simulink model "SchlossBox"  (R2017b)
settings: Solver=FixedStepAuto  StartTime=0.0  StopTime=10.0  RelTol=1e-3
PreLoadFcn:
  | waijung.modelPreload; % Required for working with Waijung Blockset. Do not remove.
undefined symbols (not defined in the file): Blocking, HSEOSC, Link, LQFP100, Non, ST, STM32F407VG
libraries: stm32f4_canbus_lib x8, simulink x6, stm32f4_io_lib x4, stm32f4_device_config_lib x1
CloseFcn:
  | waijung.modelClose; % Required for working with Waijung Blockset. Do not remove.
settings Model: Creator=labuser  LastModifiedBy=labuser
settings OptimizationCC: DefaultParameterBehavior=Inlined  PassReuseOutputArgsAs=Individual arguments
settings DebuggingCC: ParameterTunabilityLossMsg=error
settings HardwareCC: ProdBitPerPointer=32  ProdBitPerSizeT=32  ProdBitPerPtrDiffT=32  ProdLargestAtomicFloat=None  ProdIntDivRoundTo=Undefined  ProdWordSize=32  ProdHWDeviceType=ARM Compatible->Cortex - M4  TargetEndianess=LittleEndian  TargetHWDeviceType=ARM Compatible->Cortex - M4
settings SFSimCC: MATLABDynamicMemAlloc=off
settings RTWCC: SystemTargetFile=stm32f4.tlc  GenerateMakefile=off  TemplateMakefile=ert_default_tmf  Description=STM32F4 Target  GenerateReport=on  IncludeHyperlinkInReport=on  LaunchReport=on  GenerateTraceInfo=on  GenerateTraceReport=on  GenerateTraceReportSl=on  GenerateTraceReportSf=on  GenerateTraceReportEml=on
settings CodeAppCC: ForceParamTrailComments=on  IgnoreCustomStorageClasses=off  OperatorAnnotations=on  SimulinkDataObjDesc=on  SFDataObjDesc=on  InsertBlockDesc=on
settings STFCustomTargetCC: TargetLangStandard=C99 (ISO)  MultiwordLength=256  ModelReferenceCompliant=off  CombineOutputUpdateFcns=on  ERTCustomFileBanners=on  SupportContinuousTime=off  SupportNonInlinedSFcns=off  RemoveResetFunc=on  MATLABClassNameForMDSCustomization=Simulink.SoftwareTarget.ERTCustomization  GRTInterface=off  SystemTargetFile=stm32f4.tlc
settings ERTTargetCC: TargetLangStandard=C99 (ISO)  ModelReferenceCompliant=off  ParMdlRefBuildCompliant=off  CompOptLevelCompliant=off  ConcurrentExecutionCompliant=off  ModelStepFunctionPrototypeControlCompliant=off  CPPClassGenCompliant=off  UseToolchainInfoCompliant=off  InlinedParameterPlacement=NonHierarchical  ERTSrcFileBannerTemplate=stm32f4_code_template.cgt  ERTHdrFileBannerTemplate=stm32f4_code_template.cgt  ERTDataSrcFileTemplate=stm32f4_code_template.cgt  ERTDataHdrFileTemplate=stm32f4_code_template.cgt  ERTCustomFileTemplate=stm32f4_file_process.tlc

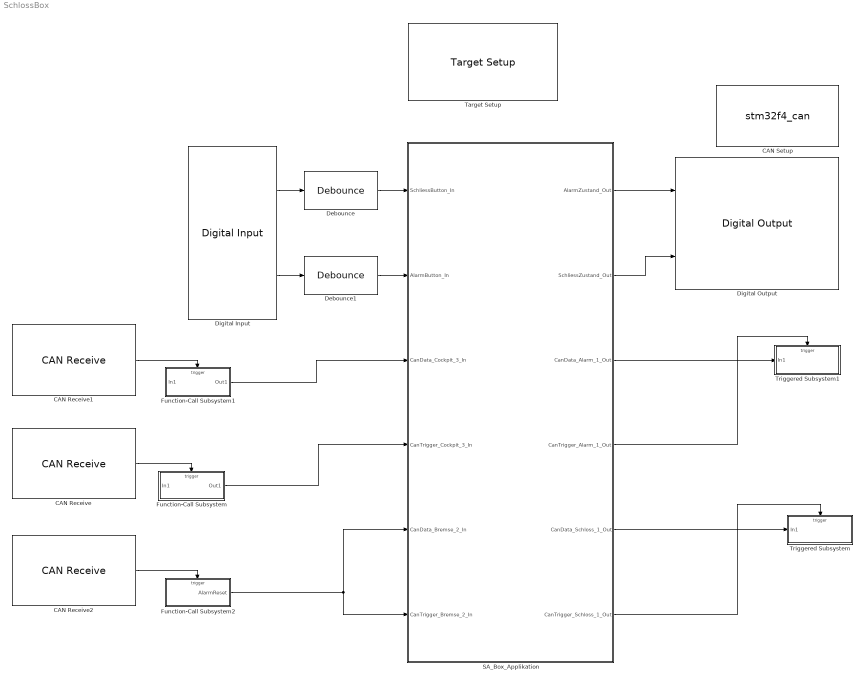
== system SchlossBox ==
  CAN Receive : stm32f4_canbus_lib/CAN Receive  conf=Rx  canmodule=1  idtype=Standard  filtertype=Specific  id=18  idmask=0  enableisr=on  usedlc=off  datatype=single  data0type=uint32  data1type=uint32  data2type=Not used  data3type=Not used  data4type=Not used  data5type=Not used  data6type=Not used  data7type=Not used  buffersize=8  sampletime=-1  sampletimestr=-1  blockid=CANReceive  inputarray=[]  inputlabelarray={}  outputarray=[7]  outputlabelarray={'Call ISR' }  compat=0  confstr="[\"Standard\",\"Specific\",\"18\",\"0\",\"off\",\"uint32\",\"uint32\",\"Not used\",\"Not used\",\"Not used\",\"Not used\",\"Not used\",\"Not used\",\"8\",\"240\",\"0\",\"FFE0\",\"4\"]"
      settings: SourceProductName=Waijung Blockset
  CAN Receive1 : stm32f4_canbus_lib/CAN Receive  conf=Rx  canmodule=1  idtype=Standard  filtertype=Specific  id=18  idmask=0  enableisr=on  usedlc=off  datatype=single  data0type=uint32  data1type=uint32  data2type=Not used  data3type=Not used  data4type=Not used  data5type=Not used  data6type=Not used  data7type=Not used  buffersize=8  sampletime=-1  sampletimestr=-1  blockid=CANReceive1  inputarray=[]  inputlabelarray={}  outputarray=[7]  outputlabelarray={'Call ISR' }  compat=0  confstr="[\"Standard\",\"Specific\",\"18\",\"0\",\"off\",\"uint32\",\"uint32\",\"Not used\",\"Not used\",\"Not used\",\"Not used\",\"Not used\",\"Not used\",\"8\",\"240\",\"0\",\"FFE0\",\"4\"]"
      settings: SourceProductName=Waijung Blockset
  CAN Receive2 : stm32f4_canbus_lib/CAN Receive  conf=Rx  canmodule=1  idtype=Standard  filtertype=Specific  id=12  idmask=0  enableisr=on  usedlc=off  datatype=single  data0type=uint32  data1type=uint32  data2type=Not used  data3type=Not used  data4type=Not used  data5type=Not used  data6type=Not used  data7type=Not used  buffersize=8  sampletime=-1  sampletimestr=-1  blockid=CANReceive1  inputarray=[]  inputlabelarray={}  outputarray=[7]  outputlabelarray={'Call ISR' }  compat=0  confstr="[\"Standard\",\"Specific\",\"12\",\"0\",\"off\",\"uint32\",\"uint32\",\"Not used\",\"Not used\",\"Not used\",\"Not used\",\"Not used\",\"Not used\",\"8\",\"180\",\"0\",\"FFE0\",\"4\"]"
      settings: SourceProductName=Waijung Blockset
  CAN Setup : S-Function  FunctionName=stm32f4_can  Parameters=conf,canmodule,0,inputarray,outputarray,'','',confstr,sampletime,sampletimestr,blockid  SFunctionDeploymentMode=off  EnableBusSupport=off  mask(stm32f4_can){conf=Setup, canmodule=1, advance=off, bitrate_select=125000, sjw=1tq, bs1=14tq, bs2=6tq, timingconf=Prescaler, brp=16, bitrate=125000, tq=3.8095e-07, autoretransmission=Disable, remaptxpin=D1, remaprxpin=D0, sampletime=0.01, sampletimestr=-1, blockid=CANSetup, inputarray=[], inputlabelarray={}, outputarray=[], outputlabelarray={}, compat=0, confstr=["125000","16","D","1","D","0","1tq","14tq","6tq","ENABLE"], presc=16, txportstr=D, txpinstr=1, rxportstr=D, rxpinstr=0, lastmodule=1}
      mask prompts: conf "Configuration"; canmodule "CAN Module"; advance "Advance configuration"; bitrate_select "Baud rate (bps)"; sjw "Resync Jump Width (SJW)"; bs1 "Bit segment 1 (BS1) + PROP_SEG"; bs2 "Bit segment 2 (BS2)"; timingconf "Adjust"; brp "Baud rate prescaler (BRP)"; bitrate "Baud rate (bps)"; tq "Time Quantum (Second), tq"; autoretransmission "Auto Re-transmission"; remaptxpin "CAN Tx pin"; remaprxpin "CAN Rx pin"; sampletime "Sample time (sec)"; sampletimestr "Compiled sample time (sec) in string"; inputarray "Input port"; inputlabelarray "Input port label"; outputarray "Output port"; outputlabelarray "Output port label"; compat "Compatibility (Reserved for future use)"; confstr "Configuration String"; presc "Prescale"; txportstr "Tx port string"; txpinstr "Tx pin string"; rxportstr "Rx port string"; rxpinstr "Rx pin string"; lastmodule "Last module selected"
      mask help:
      | This block setups CAN Module.
      |
      | Auto Re-transmission,
      |  - Enable: The CAN hardware will automatically retransmit the message until it has been
      | successfully transmitted according to the CAN standard.
      |  - Disable: A message will be transmitted only once, independently of the transmission result
      | (successful, error or arbitration lost).
      mask init:
      | stm32f4_can_callback('init');
      mask Help: web(fullfile(waijungdocroot,'stm32f4_can_setup.htm'), '-browser')
      mask TypeOptions conf: Setup
      mask TypeOptions canmodule: 1 | 2
      mask Callback canmodule: stm32f4_can_callback('canmodule');
      mask Callback advance: stm32f4_can_callback('advance');
      mask TypeOptions bitrate_select: 125000 | 250000 | 500000 | 1000000
      mask Callback bitrate_select: stm32f4_can_callback('bitrate_select');
      mask TypeOptions sjw: 1tq | 2tq | 3tq | 4tq
      mask TypeOptions bs1: 1tq | 2tq | 3tq | 4tq | 5tq | 6tq | 7tq | 8tq | 9tq | 10tq | 11tq | 12tq | 13tq | 14tq | 15tq | 16tq
      mask Callback bs1: stm32f4_can_callback('timingconf');
      mask TypeOptions bs2: 1tq | 2tq | 3tq | 4tq | 5tq | 6tq | 7tq | 8tq
      mask Callback bs2: stm32f4_can_callback('timingconf');
      mask TypeOptions timingconf: Prescaler | Baudrate
      mask Callback timingconf: stm32f4_can_callback('timingconf');
      mask Callback brp: stm32f4_can_callback('timingconf');
      mask Callback bitrate: stm32f4_can_callback('timingconf');
      mask TypeOptions autoretransmission: Enable | Disable
      mask TypeOptions remaptxpin: Not used | A12 | B9 | D1
      mask Callback remaptxpin: stm32f4_can_callback('remaptxpin');
      mask TypeOptions remaprxpin: Not used | A11 | B8 | D0
      mask Callback remaprxpin: stm32f4_can_callback('remaprxpin');
      mask Callback sampletime: stm32f4_can_callback('sampletime');
      mask Callback sampletimestr: stm32f4_can_callback('sampletimestr');
      mask Callback blockid: stm32f4_can_callback('blockid');
      mask Display: text(0.5, 0.5, 'CAN1_Setup\nSpeed (bps): 125000\nTx/Rx pin: D1/D0','ver','middle','hor','center');
  Debounce : stm32f4_io_lib/Debounce  mode=Normal  prescale=4  debounce=4
      settings: SourceProductName=Waijung Blockset
  Debounce1 : stm32f4_io_lib/Debounce  mode=Normal  prescale=4  debounce=4
      settings: SourceProductName=Waijung Blockset
  Digital Input : stm32f4_io_lib/Digital Input  port=C  speed=100  porttype=None  porttypestr=NOPULL  use_pin0=on  use_pin1=on  use_pin2=off  use_pin3=off  use_pin4=off  use_pin5=off  use_pin6=off  use_pin7=off  use_pin8=off  use_pin9=off  use_pin10=off  use_pin11=off  use_pin12=off  use_pin13=off  use_pin14=off  use_pin15=off  pinstr=GPIO_Pin_0 | GPIO_Pin_1  usedpinarray="[1  1  0  0  0  0  0  0  0  0  0  0  0  0  0  0]"  bitbandingstr=|  sampletime=-1  sampletimestr=-1  blockid=DigitalInput  enablecustomportlabel=off  glabalinit=off  cinputportlabel=In1, In2  coutputportlabel=Out1, Out2
      | #define DigitalInput_C0 Peripheral_BB(GPIOC->IDR, 0)  /* Output pin */
      | #define DigitalInput_C1 Peripheral_BB(GPIOC->IDR, 1)  /* Output pin */
      settings: SourceProductName=Waijung Blockset
  Digital Output : stm32f4_io_lib/Digital Output  use_bitband=on  port=C  speed=100  porttype=Push Pull  porttypestr=PP  use_pin0=off  use_pin1=off  use_pin2=on  use_pin3=on  use_pin4=off  use_pin5=off  use_pin6=off  use_pin7=off  use_pin8=off  use_pin9=off  use_pin10=off  use_pin11=off  use_pin12=off  use_pin13=off  use_pin14=off  use_pin15=off  pinstr=GPIO_Pin_2 | GPIO_Pin_3  usedpinarray="[0  0  1  1  0  0  0  0  0  0  0  0  0  0  0  0]"  bitbandingstr=|  sampletime=-1  sampletimestr=-1  blockid=DigitalOutput  enablecustomportlabel=off  globalinit=off  cinputportlabel=In1, In2  coutputportlabel=0
      | #define DigitalOutput_C2 Peripheral_BB(GPIOC->ODR, 2)  /* Output pin */
      | #define DigitalOutput_C3 Peripheral_BB(GPIOC->ODR, 3)  /* Output pin */
      settings: SourceProductName=Waijung Blockset
  Function-Call Subsystem : Subsystem  TreatAsAtomicUnit=on
  Function-Call Subsystem1 : Subsystem  TreatAsAtomicUnit=on
  Function-Call Subsystem2 : Subsystem  TreatAsAtomicUnit=on
  SA_Box_Applikation : Subsystem
  Target Setup : stm32f4_device_config_lib/Target Setup  Priority=100  compiler=GNU ARM  previous_compiler=GNU ARM  mcu=STM32F407VG (LQFP100)  mcustr=STM32F407VG  clockconfig=HSEOSC-8MHz  system_stm32f4xx_c_path=C:\waijung17_03a\targets\stm32f4_target\stm32f4\utils\system_stm32f4xx_default\STM32F40_41xxx\hseosc8mhz  showmemoryconfiguration=off  stacksize=0x2000  heapsize=0x2000  enableautocompiledownload=on  fullchiperase=off  programmerinterface=ST-Link  editctrlstr=on  compilercontrolstr=$(patsubst %, -I%, .) -mcpu=cortex-m4 -mthumb -mthumb-interwork -mfloat-abi=hard -mfpu=fpv4-sp-d16 -ffast-math -Wall -Wextra -Ofast  assemblercontrolstr=$(patsubst %, -I%, .) -mcpu=cortex-m4 -mthumb -mthumb-interwork -mfloat-abi=hard -mfpu=fpv4-sp-d16 -ffast-math -Wall -Wextra -Ofast -Wa,-amhls=$(<:.s=.lst) -D__STACK_SIZE=$(STACK_SIZE) -D__HEAP_SIZE=$(HEAP_SIZE)  linkercontrolstr=-T$(LD_SCRIPT) -g -Wl,-Map=$(MAP),--cref,--no-warn-mismatch -mcpu=cortex-m4 -mthumb -mthumb-interwork -mfloat-abi=hard -mfpu=fpv4-sp-d16 -specs=nosys.specs  runafterdownload=on  execprofile=None  profileruart=3  profilerbaud=500000  profilertxpin=D8  profilerinitstr=0.01,168000000,1680000,500000,0  manualsetsampletime=off  sampletime=0.01  blockid=TargetSetup  systickreloadvalue=1680000  hseval=8000000  lastprofileruart=3  hclk=168000000  flashorigin=0x8000000  flashlength=1024k  ramorigin=0x20000000  ramlength=128k  useextram=off
      settings: SourceProductName=Waijung Blockset
  Triggered Subsystem : Subsystem  TreatAsAtomicUnit=on
  Triggered Subsystem1 : Subsystem  TreatAsAtomicUnit=on
  wires:
  Function-Call Subsystem2/1(AlarmReset) -> SA_Box_Applikation/5(CanData_Bremse_2_In), SA_Box_Applikation/6(CanTrigger_Bremse_2_In)
  SA_Box_Applikation/5(CanData_Schloss_1_Out) -> Triggered Subsystem/1(In1)
  CAN Receive/1 -> Function-Call Subsystem/Trigger
  Function-Call Subsystem/1(Out1) -> SA_Box_Applikation/4(CanTrigger_Cockpit_3_In)
  CAN Receive1/1 -> Function-Call Subsystem1/Trigger
  Function-Call Subsystem1/1(Out1) -> SA_Box_Applikation/3(CanData_Cockpit_3_In)
  Digital Input/2 -> Debounce1/1
  SA_Box_Applikation/3(CanData_Alarm_1_Out) -> Triggered Subsystem1/1(In1)
  SA_Box_Applikation/2(SchliessZustand_Out) -> Digital Output/2
  SA_Box_Applikation/1(AlarmZustand_Out) -> Digital Output/1
  Digital Input/1 -> Debounce/1
  Debounce/1 -> SA_Box_Applikation/1(SchliessButton_In)
  Debounce1/1 -> SA_Box_Applikation/2(AlarmButton_In)
  SA_Box_Applikation/4(CanTrigger_Alarm_1_Out) -> Triggered Subsystem1/Trigger
  SA_Box_Applikation/6(CanTrigger_Schloss_1_Out) -> Triggered Subsystem/Trigger
  CAN Receive2/1 -> Function-Call Subsystem2/Trigger

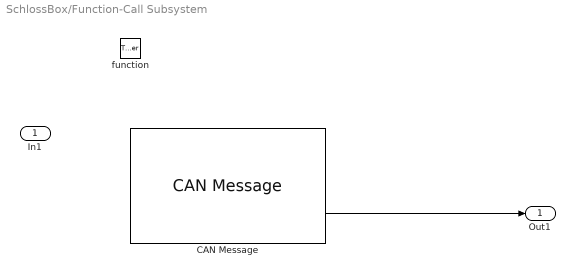
== system SchlossBox/Function-Call Subsystem ==
  In1 : Inport
  function : TriggerPort  TriggerType=function-call  VariantControl=Variant
  CAN Message : stm32f4_canbus_lib/CAN Message  conf=Msg  canmodule=1  usedlc=off  datatype=double  data0type=uint8  data1type=Not used  data2type=Not used  data3type=Not used  data4type=Not used  data5type=Not used  data6type=Not used  data7type=Not used  sampletime=-1  sampletimestr=-1  blockid=FunctionCallSubsystemCANMessage  inputarray=[]  inputlabelarray={}  outputarray=[ 7, 3]  outputlabelarray={'ID', 'D0 (uint8)' }  compat=0  confstr="[\"off\",\"uint8\",\"Not used\",\"Not used\",\"Not used\",\"Not used\",\"Not used\",\"Not used\",\"Not used\"]"
      settings: SourceProductName=Waijung Blockset
  Out1 : Outport
  wires:
  CAN Message/2 -> Out1/1

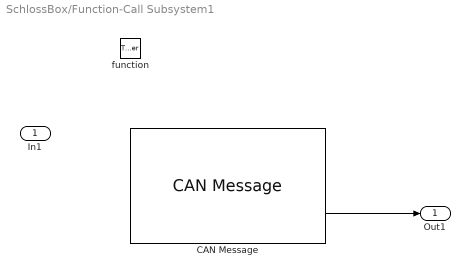
== system SchlossBox/Function-Call Subsystem1 ==
  In1 : Inport
  function : TriggerPort  TriggerType=function-call  VariantControl=Variant
  CAN Message : stm32f4_canbus_lib/CAN Message  conf=Msg  canmodule=1  usedlc=off  datatype=double  data0type=uint8  data1type=Not used  data2type=Not used  data3type=Not used  data4type=Not used  data5type=Not used  data6type=Not used  data7type=Not used  sampletime=-1  sampletimestr=-1  blockid=FunctionCallSubsystem1CANMessage  inputarray=[]  inputlabelarray={}  outputarray=[ 7, 3]  outputlabelarray={'ID', 'D0 (uint8)' }  compat=0  confstr="[\"off\",\"uint8\",\"Not used\",\"Not used\",\"Not used\",\"Not used\",\"Not used\",\"Not used\",\"Not used\"]"
      settings: SourceProductName=Waijung Blockset
  Out1 : Outport
  wires:
  CAN Message/2 -> Out1/1

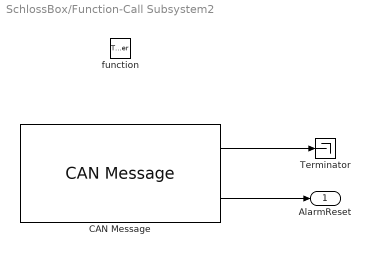
== system SchlossBox/Function-Call Subsystem2 ==
  function : TriggerPort  TriggerType=function-call  VariantControl=Variant
  CAN Message : stm32f4_canbus_lib/CAN Message  conf=Msg  canmodule=1  usedlc=off  datatype=double  data0type=uint8  data1type=Not used  data2type=Not used  data3type=Not used  data4type=Not used  data5type=Not used  data6type=Not used  data7type=Not used  sampletime=-1  sampletimestr=-1  blockid=FunctionCallSubsystem1CANMessage  inputarray=[]  inputlabelarray={}  outputarray=[ 7, 3]  outputlabelarray={'ID', 'D0 (uint8)' }  compat=0  confstr="[\"off\",\"uint8\",\"Not used\",\"Not used\",\"Not used\",\"Not used\",\"Not used\",\"Not used\",\"Not used\"]"
      settings: SourceProductName=Waijung Blockset
  Terminator : Terminator
  AlarmReset : Outport
  wires:
  CAN Message/1 -> Terminator/1
  CAN Message/2 -> AlarmReset/1

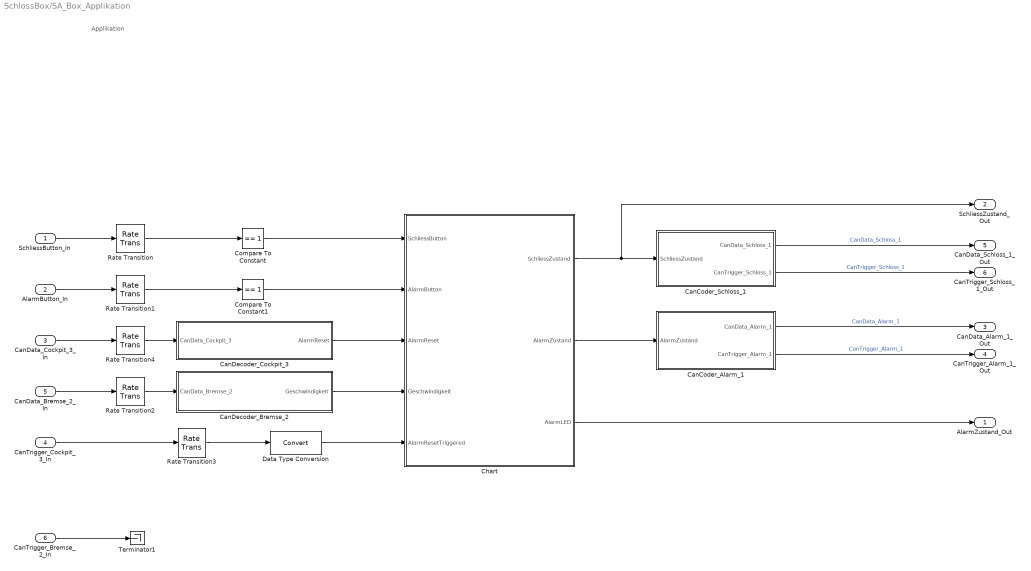
== system SchlossBox/SA_Box_Applikation ==
  note: Applikation
  SchliessButton_In : Inport
  AlarmButton_In : Inport  Port=2
  CanData_Cockpit_3_In : Inport  Port=3
  CanTrigger_Cockpit_3_In : Inport  Port=4
  CanData_Bremse_2_In : Inport  Port=5
  CanTrigger_Bremse_2_In : Inport  Port=6
  CanCoder_Alarm_1 : Subsystem
  CanCoder_Schloss_1 : Subsystem
  CanDecoder_Bremse_2 : Subsystem
  CanDecoder_Cockpit_3 : Subsystem
  Chart : Stateflow chart  TreatAsAtomicUnit=on
  Compare To Constant : simulink/Logic and Bit Operations/Compare To Constant  relop===  const=1  OutDataTypeStr=uint8
  Compare To Constant1 : simulink/Logic and Bit Operations/Compare To Constant  relop===  const=1  OutDataTypeStr=uint8
  Data Type Conversion : DataTypeConversion
  Rate Transition{,1..4} (5 alike) : RateTransition  Deterministic=off  OutPortSampleTimeOpt=Inherit
  Terminator1 : Terminator
  AlarmZustand_Out : Outport
  SchliessZustand_Out : Outport  Port=2
  CanData_Alarm_1_Out : Outport  Port=3
  CanTrigger_Alarm_1_Out : Outport  Port=4
  CanData_Schloss_1_Out : Outport  Port=5
  CanTrigger_Schloss_1_Out : Outport  Port=6
  wires:
  CanCoder_Schloss_1/1(CanData_Schloss_1) -> CanData_Schloss_1_Out/1  "CanData_Schloss_1"
  CanCoder_Alarm_1/1(CanData_Alarm_1) -> CanData_Alarm_1_Out/1  "CanData_Alarm_1"
  CanCoder_Alarm_1/2(CanTrigger_Alarm_1) -> CanTrigger_Alarm_1_Out/1  "CanTrigger_Alarm_1"
  CanCoder_Schloss_1/2(CanTrigger_Schloss_1) -> CanTrigger_Schloss_1_Out/1  "CanTrigger_Schloss_1"
  CanDecoder_Cockpit_3/1(AlarmReset) -> Chart/3(AlarmReset)
  CanDecoder_Bremse_2/1(Geschwindigkeit) -> Chart/4(Geschwindigkeit)
  Chart/2(AlarmZustand) -> CanCoder_Alarm_1/1(AlarmZustand)
  CanData_Cockpit_3_In/1 -> Rate Transition4/1
  SchliessButton_In/1 -> Rate Transition/1
  CanData_Bremse_2_In/1 -> Rate Transition2/1
  AlarmButton_In/1 -> Rate Transition1/1
  CanTrigger_Bremse_2_In/1 -> Terminator1/1
  Chart/3(AlarmLED) -> AlarmZustand_Out/1
  Chart/1(SchliessZustand) -> SchliessZustand_Out/1, CanCoder_Schloss_1/1(SchliessZustand)
  Rate Transition4/1 -> CanDecoder_Cockpit_3/1(CanData_Cockpit_3)
  Rate Transition2/1 -> CanDecoder_Bremse_2/1(CanData_Bremse_2)
  Rate Transition3/1 -> Data Type Conversion/1
  CanTrigger_Cockpit_3_In/1 -> Rate Transition3/1
  Data Type Conversion/1 -> Chart/5(AlarmResetTriggered)
  Rate Transition/1 -> Compare To Constant/1
  Rate Transition1/1 -> Compare To Constant1/1
  Compare To Constant/1 -> Chart/1(SchliessButton)
  Compare To Constant1/1 -> Chart/2(AlarmButton)

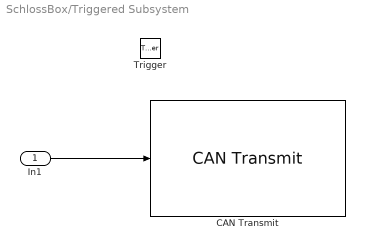
== system SchlossBox/Triggered Subsystem ==
  In1 : Inport
  Trigger : TriggerPort  VariantControl=Variant
  CAN Transmit : stm32f4_canbus_lib/CAN Transmit  conf=Tx  canmodule=1  transfer=Non-Blocking  timeout=0.005  idtype=Standard  specificid=on  id=25  specificdlc=on  dlc=2  enablestatus=off  datatype=single  data0type=int16  data1type=Not used  data2type=Not used  data3type=Not used  data4type=Not used  data5type=Not used  data6type=Not used  data7type=Not used  inputarray=[ 4]  inputlabelarray={ 'D0 (int16)' }  outputarray=[]  outputlabelarray={}  sampletime=-1  sampletimestr=-1  blockid=TriggeredSubsystemCANTransmit  compat=0  confstr="[\"Non-Blocking\",\"0.005\",\"Standard\",\"on\",\"25\",\"on\",\"2\",\"off\",\"int16\",\"Not used\",\"Not used\",\"Not used\",\"Not used\",\"Not used\",\"Not used\",\"Not used\"]"
      settings: SourceProductName=Waijung Blockset
  wires:
  In1/1 -> CAN Transmit/1

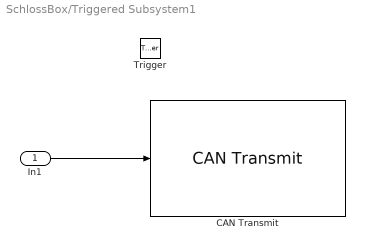
== system SchlossBox/Triggered Subsystem1 ==
  In1 : Inport
  Trigger : TriggerPort  VariantControl=Variant
  CAN Transmit : stm32f4_canbus_lib/CAN Transmit  conf=Tx  canmodule=1  transfer=Non-Blocking  timeout=0.005  idtype=Standard  specificid=on  id=20  specificdlc=on  dlc=2  enablestatus=off  datatype=single  data0type=int16  data1type=Not used  data2type=Not used  data3type=Not used  data4type=Not used  data5type=Not used  data6type=Not used  data7type=Not used  inputarray=[ 4]  inputlabelarray={ 'D0 (int16)' }  outputarray=[]  outputlabelarray={}  sampletime=-1  sampletimestr=-1  blockid=TriggeredSubsystem1CANTransmit  compat=0  confstr="[\"Non-Blocking\",\"0.005\",\"Standard\",\"on\",\"20\",\"on\",\"2\",\"off\",\"int16\",\"Not used\",\"Not used\",\"Not used\",\"Not used\",\"Not used\",\"Not used\",\"Not used\"]"
      settings: SourceProductName=Waijung Blockset
  wires:
  In1/1 -> CAN Transmit/1

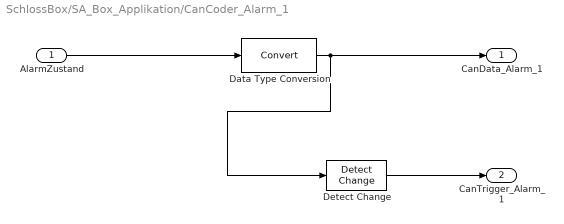
== system SchlossBox/SA_Box_Applikation/CanCoder_Alarm_1 ==
  AlarmZustand : Inport
  Data Type Conversion : DataTypeConversion
  Detect Change : simulink/Logic and Bit Operations/Detect Change  vinit=0  OutDataTypeStr=uint8
  CanData_Alarm_1 : Outport
  CanTrigger_Alarm_1 : Outport  Port=2
  wires:
  Detect Change/1 -> CanTrigger_Alarm_1/1
  AlarmZustand/1 -> Data Type Conversion/1
  Data Type Conversion/1 -> Detect Change/1, CanData_Alarm_1/1

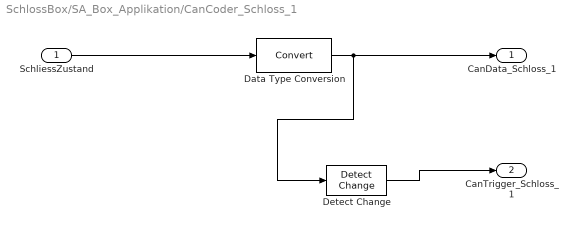
== system SchlossBox/SA_Box_Applikation/CanCoder_Schloss_1 ==
  SchliessZustand : Inport
  Data Type Conversion : DataTypeConversion
  Detect Change : simulink/Logic and Bit Operations/Detect Change  vinit=0  OutDataTypeStr=uint8
  CanData_Schloss_1 : Outport
  CanTrigger_Schloss_1 : Outport  Port=2
  wires:
  SchliessZustand/1 -> Data Type Conversion/1
  Data Type Conversion/1 -> Detect Change/1, CanData_Schloss_1/1
  Detect Change/1 -> CanTrigger_Schloss_1/1

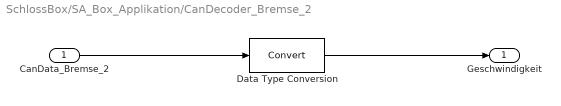
== system SchlossBox/SA_Box_Applikation/CanDecoder_Bremse_2 ==
  CanData_Bremse_2 : Inport
  Data Type Conversion : DataTypeConversion
  Geschwindigkeit : Outport
  wires:
  CanData_Bremse_2/1 -> Data Type Conversion/1
  Data Type Conversion/1 -> Geschwindigkeit/1

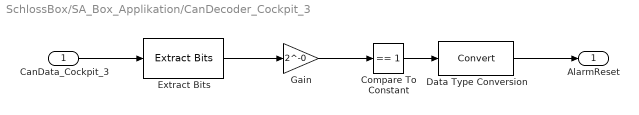
== system SchlossBox/SA_Box_Applikation/CanDecoder_Cockpit_3 ==
  CanData_Cockpit_3 : Inport
  Compare To Constant : simulink/Logic and Bit Operations/Compare To Constant  relop===  const=1  OutDataTypeStr=boolean
  Data Type Conversion : DataTypeConversion
  Extract Bits : simulink/Logic and Bit Operations/Extract Bits  bitsToExtract=Range of bits  numBits=8  bitIdxRange=[0]  outScalingMode=Preserve fixed-point scaling
  Gain : Gain  Gain=2^-0
  AlarmReset : Outport
  wires:
  Compare To Constant/1 -> Data Type Conversion/1
  CanData_Cockpit_3/1 -> Extract Bits/1
  Extract Bits/1 -> Gain/1
  Gain/1 -> Compare To Constant/1
  Data Type Conversion/1 -> AlarmReset/1

== stateflow chart SchlossBox/SA_Box_Applikation/Chart ==
  state ALARM [parallel]
    entry:
    SchliessZustand=0;
    AlarmZustand=0;
    AlarmLED=0;
    settings: executionOrder=2
    state Alarm [parallel]
      settings: executionOrder=1
      state ALARM_AUS
        entry:
        AlarmZustand=0;
        AlarmLED=0;
      state ALARM_AUSSCHALTBAR
      state TRIGGER_OFF
        entry:
        AlarmZustand=0;
        during:
        AlarmLED=blinken;
      state TRIGGER_ON
        entry:
        AlarmZustand=1;
        AlarmLED=1;
      state Knopf_Gedrueckt
      (default) -> ALARM_AUS
      ALARM_AUSSCHALTBAR -> ALARM_AUS : [AlarmReset==1]
      TRIGGER_ON -> ALARM_AUSSCHALTBAR : [SchliessZustand==0]
      ALARM_AUS -> TRIGGER_OFF : [Geschwindigkeit==0 && SchliessZustand==1]
      TRIGGER_OFF -> ALARM_AUS [order 2] : [SchliessZustand==0 || Geschwindigkeit > 0]
      TRIGGER_OFF -> Knopf_Gedrueckt [order 1] : [AlarmButton==1]
      Knopf_Gedrueckt -> TRIGGER_ON : [AlarmButton==0]
    state BLINKEN [parallel]
      entry:
      blinken=0;
      settings: executionOrder=2
      state LED_EIN
        entry:
        blinken=1;
      state LED_AUS
        entry:
        blinken=0;
      (default) -> LED_EIN
      LED_AUS -> LED_EIN : after(1,sec)
      LED_EIN -> LED_AUS : after(1,sec)
  state Schliessanlage [parallel]
    entry:
    SchliessZustand=1;
    AlarmZustand=0;
    AlarmLED=0;
    settings: executionOrder=1
    state OFFEN
      entry:
      SchliessZustand=0;
    state GESCHLOSSEN
      entry:
      SchliessZustand=1;
    state Betaetigungsdauer
    state Betaetigungsdauer1
    (default) -> GESCHLOSSEN
    Betaetigungsdauer -> GESCHLOSSEN : [SchliessButton==1]
    OFFEN -> Betaetigungsdauer : [SchliessButton==0]
    GESCHLOSSEN -> Betaetigungsdauer1 : [SchliessButton==0]
    Betaetigungsdauer1 -> OFFEN : [SchliessButton==1]
  data: blinken local uint8; SchliessButton input; AlarmButton input; SchliessZustand output uint8; AlarmZustand output uint8; AlarmReset input; Geschwindigkeit input; AlarmLED output uint8; AlarmResetTriggered input boolean
  events: AlarmResetUpdated local FUNCTION_CALL_EVENT
